simulink model "Program_1_SIR_China 2"  (R2019b)
settings: Solver=FixedStepAuto  StartTime=0.0  StopTime=90  FixedStep=0.001  RelTol=1e-9  AbsTol=1e-9
values from neighbouring files (symbols this model uses):
  a = 0.5    [Main_China_SIR_Program_1.m]
  beta = 1.17386114378623    (= 1.17386114379)    [Main_China_SIR_Program_1.m]
  gamma1 = 0.65905784176993    (= 0.65905784177)    [Main_China_SIR_Program_1.m]
  gamma2 = 0.922873642259164    (= 0.922873642259)    [Main_China_SIR_Program_1.m]
  gamma3 = 1.06040119904744    (= 1.06040119905)    [Main_China_SIR_Program_1.m]
  I0 = 1    [Main_China_SIR_Program_1.m]
  P = 11*10^6    (= 11000000)    [Main_China_SIR_Program_1.m]
  R0 = 0    [Main_China_SIR_Program_1.m]
  zeta1 = -0.251586911587193    (= -0.251586911587)    [Main_China_SIR_Program_1.m]
  zeta2 = -0.124211246181375    (= -0.124211246181)    [Main_China_SIR_Program_1.m]
  zeta3 = -0.311839590070327    (= -0.31183959007)    [Main_China_SIR_Program_1.m]
libraries: fuzblock x3
settings Model: OrderedModelArguments=off  Creator=ismae  LastModifiedBy=ismae
settings SolverCC: SolverResetMethod=Robust

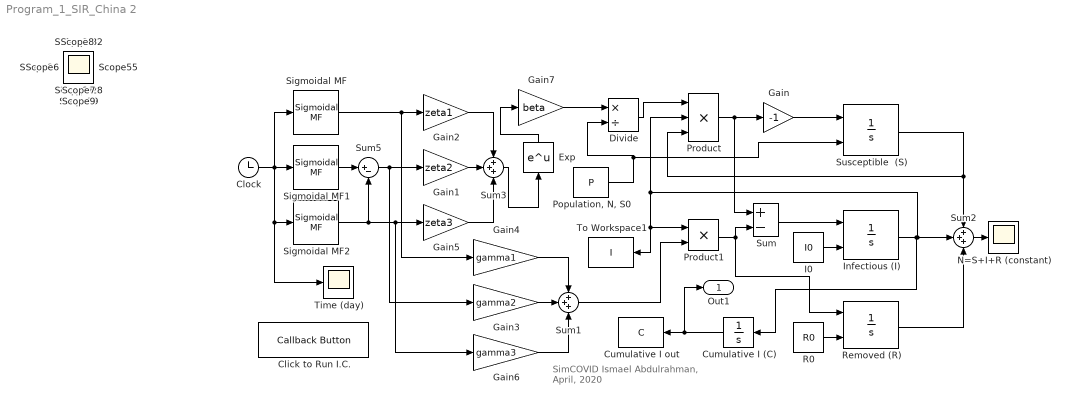
== system Program_1_SIR_China 2 ==
  note: SimCOVID
      | Ismael Abdulrahman, April, 2020
  Click to Run I.C. : CallbackButton  Description=Run this callback button first to evaluate the initial values for the parameters
      settings: ClickFcn=|
      | P   = 11*10^6; % Population, Susceptible, N, S0
      | I0  = 1;       % Initial value for "Infectious"
      | R0  = 0;       % Initial value for "Removed"
      | st1 = 28;      % starting time 1 (step time)
      | st2 = 44;      % starting time 2 (step time)
      | a   = 0.5;     % parameter of the sigmoid function
      | %==========================================================================
      | %%%%% These are the final values from the optimization obtained by Simulink
      | beta    = 1.17386114378623;
      | gamma1  = 0.65905784176993;
      | gamma2  = 0.922873642259164;
      | gamma3  = 1.06040119904744;
      | zeta1   = -0.251586911587193;
      | zeta2   = -0.124211246181375;
      | zeta3   = -0.311839590070327;
      | I1  = xlsread('COVID-19-geographic-disbtribution-worldwide-2020-04-05','China','E:E');
      | I   = flip(I1);
      | C   = cumsum(I);               % Cumulative sum of I
      | t   = 1:length(C);
      | xy  = [t' C];
      | xy0 = [t' I];
  Clock : Clock
  Cumulative I (C) : Integrator
  Cumulative I out : ToWorkspace  VariableName=C  SaveFormat=Timeseries  SampleTime=-1
      settings: Save2DSignal=2-D array (concatenate along first dimension)
  Divide : Product  Inputs=*/
  Exp : Math  SignedPower=off  SaturateOnIntegerOverflow=on
  Gain : Gain  Gain=-1
  Gain1 : Gain  Gain=zeta2
  Gain2 : Gain  Gain=zeta1
  Gain3 : Gain  Gain=gamma2
  Gain4 : Gain  Gain=gamma1
  Gain5 : Gain  Gain=zeta3
  Gain6 : Gain  Gain=gamma3
  Gain7 : Gain  Gain=beta
  I0 : Constant  Value=I0
  Infectious (I) : Integrator  InitialConditionSource=external
  N=S+I+R (constant) : Scope
  "Population, N, S0" : Constant  Value=P
  Product : Product  Inputs=3
  Product1 : Product
  R0 : Constant  Value=R0
  Removed (R) : Integrator  InitialConditionSource=external
  Sigmoidal MF : fuzblock/Membership  Functions/Sigmoidal MF  a=-a  c=st1
      settings: SourceProductName=Fuzzy Logic Toolbox  SourceProductBaseCode=FL
  Sigmoidal MF1 : fuzblock/Membership  Functions/Sigmoidal MF  a=a  c=st1
      settings: SourceProductName=Fuzzy Logic Toolbox  SourceProductBaseCode=FL
  Sigmoidal MF2 : fuzblock/Membership  Functions/Sigmoidal MF  a=a  c=st2
      settings: SourceProductName=Fuzzy Logic Toolbox  SourceProductBaseCode=FL
  Sum : Sum  Inputs=+-
  Sum1 : Sum  Inputs=+++
  Sum2 : Sum  Inputs=+++
  Sum3 : Sum  Inputs=+++
  Sum5 : Sum  Inputs=|+-
  Susceptible  (S) : Integrator  InitialConditionSource=external  InitialCondition=10000
  Time (day) : Scope
  To Workspace1 : ToWorkspace  VariableName=I  SaveFormat=Timeseries  SampleTime=-1
      settings: Save2DSignal=2-D array (concatenate along first dimension)
  Out1 : Outport
  Scope{,1..32} (33 alike) : Scope
  wires:
  Product/1 -> Gain/1, Sum/1
  Divide/1 -> Product/1
  Sum/1 -> Infectious (I)/1
  I0/1 -> Infectious (I)/2
  "Population, N, S0"/1 -> Susceptible  (S)/2, Divide/2
  Sum2/1 -> N=S+I+R (constant)/1
  R0/1 -> Removed (R)/2
  Product1/1 -> Removed (R)/1, Sum/2
  Gain5/1 -> Sum3/3
  Gain1/1 -> Sum3/2
  Gain2/1 -> Sum3/1
  Susceptible  (S)/1 -> Product/3, Sum2/1
  Gain/1 -> Susceptible  (S)/1
  Infectious (I)/1 -> Product1/1, To Workspace1/1, Product/2, Sum2/2, Cumulative I (C)/1
  Removed (R)/1 -> Sum2/3
  Cumulative I (C)/1 -> Cumulative I out/1, Out1/1
  Sum3/1 -> Exp/1
  Exp/1 -> Gain7/1
  Sum1/1 -> Product1/2
  Sigmoidal MF/1 -> Gain4/1, Gain2/1
  Sigmoidal MF1/1 -> Sum5/1
  Gain4/1 -> Sum1/1
  Sigmoidal MF2/1 -> Gain6/1, Gain5/1, Sum5/2
  Sum5/1 -> Gain3/1, Gain1/1
  Gain7/1 -> Divide/1
  Gain6/1 -> Sum1/3
  Gain3/1 -> Sum1/2
  Clock/1 -> Sigmoidal MF/1, Sigmoidal MF1/1, Sigmoidal MF2/1, Time (day)/1
